simulink model "PID"  (R2022b)
settings: Solver=ode45  StartTime=0.0  StopTime=25  RelTol=1e-3
values from neighbouring files (symbols this model uses):
  Beq = 2.0e-6    (= 2e-06)    [parameters.m]
  Jeq = mot.J + mld.Jl / (gbox.N ^ 2)    [parameters.m]
  Kd = Kp * Td / 1.5    [parameters.m]
  Ki = Kp / Ti / 30    [parameters.m]
  Kp = deltaK * cos(delta_phi) * 2    [parameters.m]
  rads2rpm = 60/2/pi    (= 9.54929658551)    [parameters.m]
  Req = mot.R + Rs    [parameters.m]
  Tl = 1 /(3.5 * w_gc)    [parameters.m]
undefined symbols (not defined in the file or in its folder): drv, gbox, mld, mot
libraries: simulink x1
settings Model: SimulationMode=accelerator  Creator=nazanin  LastModifiedBy=nazanin
settings SolverCC: ZeroCrossAlgorithm=Adaptive
settings DebuggingCC: IgnoredZcDiagnostic=none

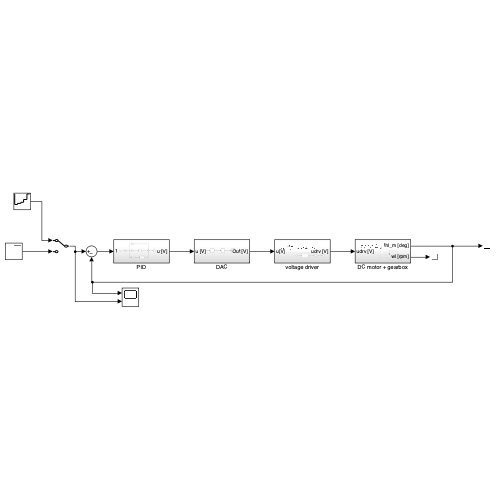
[thumbnail: Simulink's stored preview of the top-level diagram]
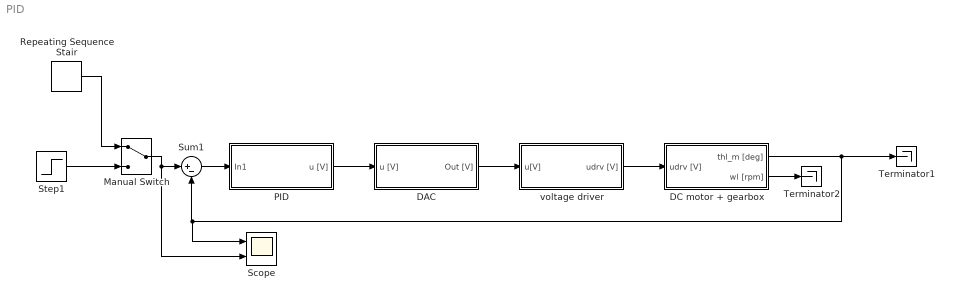
== system PID ==
  DAC : Subsystem
  DC motor + gearbox : Subsystem
  Manual Switch : ManualSwitch
  PID : Subsystem
  Repeating Sequence Stair : simulink/Sources/Repeating Sequence Stair  OutValues=[10 45 90 180 360].'  tsamp=5  OutMin=[]  OutMax=[]  OutDataTypeStr=double  OutputDataTypeScalingMode=double  OutDataType=fixdt(0,8)  ConRadixGroup=Best Precision: Vector-wise  OutScaling=2^-12
  Scope : Scope  NumInputPorts=2
  Step1 : Step  Time=0  After=70  SampleTime=0
  Sum1 : Sum  Inputs=|+-
  Terminator1 : Terminator
  Terminator2 : Terminator
  voltage driver : Subsystem
  wires:
  voltage driver/1(udrv [V]) -> DC motor + gearbox/1(udrv [V])
  DC motor + gearbox/2(wl [rpm]) -> Terminator2/1
  DAC/1(Out [V]) -> voltage driver/1(u[V])
  DC motor + gearbox/1(thl_m [deg]) -> Scope/1, Sum1/2, Terminator1/1
  Sum1/1 -> PID/1(In1)
  PID/1(u [V]) -> DAC/1(u [V])
  Step1/1 -> Manual Switch/2
  Repeating Sequence Stair/1 -> Manual Switch/1
  Manual Switch/1 -> Scope/2, Sum1/1

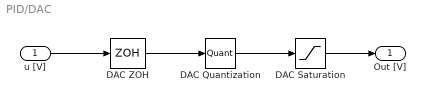
== system PID/DAC ==
  u [V] : Inport
  DAC Quantization : Quantizer  QuantizationInterval=20/(2^16 - 1)
  DAC Saturation : Saturate  UpperLimit=10  LowerLimit=-10
  DAC ZOH : ZeroOrderHold  SampleTime=0.001
  Out [V] : Outport
  wires:
  DAC Saturation/1 -> Out [V]/1
  DAC Quantization/1 -> DAC Saturation/1
  DAC ZOH/1 -> DAC Quantization/1
  u [V]/1 -> DAC ZOH/1

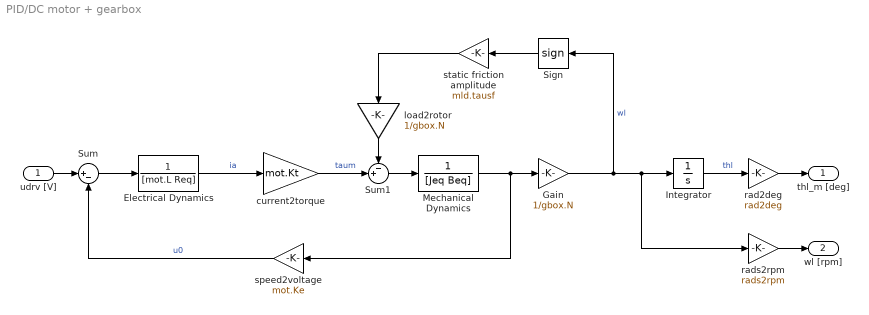
== system PID/DC motor + gearbox ==
  udrv [V] : Inport
  Electrical Dynamics : TransferFcn  Denominator=[mot.L Req]
  Gain : Gain  Gain=1/gbox.N
  Integrator : Integrator
  Mechanical Dynamics : TransferFcn  Denominator=[Jeq Beq]
  Sign : Signum  ZeroCross=off
  Sum : Sum  Inputs=|+-
  Sum1 : Sum  Inputs=-+|
  current2torque : Gain  Gain=mot.Kt
  load2rotor : Gain  Gain=1/gbox.N
  rad2deg : Gain  Gain=rad2deg
  rads2rpm : Gain  Gain=rads2rpm
  speed2voltage : Gain  Gain=mot.Ke
  static friction amplitude : Gain  Gain=mld.tausf
  thl_m [deg] : Outport
  wl [rpm] : Outport  Port=2
  wires:
  rads2rpm/1 -> wl [rpm]/1
  current2torque/1 -> Sum1/2  "taum"
  Mechanical Dynamics/1 -> Gain/1, speed2voltage/1
  Sign/1 -> static friction amplitude/1
  speed2voltage/1 -> Sum/2  "u0"
  Integrator/1 -> rad2deg/1  "thl"
  Sum/1 -> Electrical Dynamics/1
  rad2deg/1 -> thl_m [deg]/1
  udrv [V]/1 -> Sum/1
  Electrical Dynamics/1 -> current2torque/1  "ia"
  static friction amplitude/1 -> load2rotor/1
  Gain/1 -> rads2rpm/1, Integrator/1, Sign/1  "wl"
  Sum1/1 -> Mechanical Dynamics/1
  load2rotor/1 -> Sum1/1

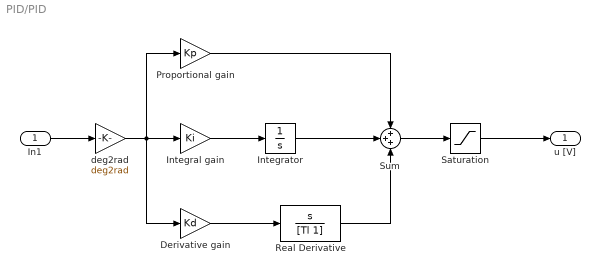
== system PID/PID ==
  In1 : Inport
  Derivative gain : Gain  Gain=Kd
  Integral gain : Gain  Gain=Ki
  Integrator : Integrator
  Proportional gain : Gain  Gain=Kp
  Real Derivative : TransferFcn  Numerator=[1 0]  Denominator=[Tl 1]
  Saturation : Saturate  UpperLimit=10  LowerLimit=-10
  Sum : Sum  Inputs=+++
  deg2rad : Gain  Gain=deg2rad
  u [V] : Outport
  wires:
  In1/1 -> deg2rad/1
  deg2rad/1 -> Derivative gain/1, Proportional gain/1, Integral gain/1
  Integral gain/1 -> Integrator/1
  Integrator/1 -> Sum/2
  Proportional gain/1 -> Sum/1
  Derivative gain/1 -> Real Derivative/1
  Sum/1 -> Saturation/1
  Saturation/1 -> u [V]/1
  Real Derivative/1 -> Sum/3

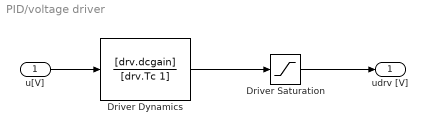
== system PID/voltage driver ==
  u[V] : Inport
  Driver Dynamics : TransferFcn  Numerator=[drv.dcgain]  Denominator=[drv.Tc 1]
  Driver Saturation : Saturate  UpperLimit=12  LowerLimit=-12
  udrv [V] : Outport
  wires:
  Driver Dynamics/1 -> Driver Saturation/1
  Driver Saturation/1 -> udrv [V]/1
  u[V]/1 -> Driver Dynamics/1
